simulink model "ES241A_MotAg2Meas"  (R2013b)
settings: Solver=FixedStepDiscrete  SolverMode=SingleTasking  StartTime=0.0  StopTime=1  FixedStep=0.002  RelTol=1e-3
undefined symbols (not defined in the file): ARCHGLBPRM_2PI_ULS_F32, FLTINJ_MOTAG2MEAS_MOTAG2MECL, MOTAG2ANSINCOSFLTFAILSTEP_CNT_U16, MOTAG2ANSINCOSFLTPASSSTEP_CNT_U16, MotAg2MeasOffs, MOTAG2MECLMAX_MOTREV_F32, MOTAG2MECLMIN_MOTREV_F32, NtcNr1, NtcSts1, sigbuilder_block, VALMAXERR_VOLTSQD_F32, VALMINERR_VOLTSQD_F32
libraries: simulink x12, NxtrLim x2, FloatToFixd x1, NxtrMath x1
(part 3 of 3)

== stateflow chart ES241A_MotAg2Meas/MotAg2Meas/MotAg2MeasPer1/MotPos_ArcTan/LimitMotAg2Meas/NormalizeMotAg2Mecl ==
  (default) -> (junction 3)
  (junction 3) -> (junction 5) : {MotAg2MeclVar=MotAg2MeclIn;}
  (junction 5) -> (junction 7) [order 2] : [MotAg2MeclVar<0]
  (junction 5) -> (junction 6) [order 1] : [MotAg2MeclVar>1]
  (junction 6) -> (junction 5) : {MotAg2MeclVar=MotAg2MeclVar-1;}
  (junction 7) -> (junction 5) : {MotAg2MeclVar=MotAg2MeclVar+1;}
  (junction 5) -> (junction 13) [order 3] : {MotAg2Mecl=MotAg2MeclVar;}
  data: MotAg2MeclIn input; MotAg2Mecl output single; MotAg2MeclVar local single

== stateflow chart ES241A_MotAg2Meas/MotAg2Meas/MotAg2MeasPer1/AnalogMsbDiagnostics/RollCnt_Qulfr_Calc/RollingCntr_Calc ==
  settings: stateMachineType=MEALY_MACHINE
  (default) -> (junction 4)
  (junction 4) -> (junction 6) [order 1] : [TestOk==1]
  (junction 6) -> (junction 36) [order 2] : {RollgCntr = PrevRollgCntr+1;}
  (junction 4) -> (junction 20) [order 2]
  (junction 6) -> (junction 36) [order 1] : [PrevRollgCntr == 255]
      | {
      | RollgCntr = 0;
      | }
  (junction 36) -> (junction 20)
  data: TestOk input; PrevRollgCntr input uint8 [0..255] =0; RollgCntr output uint8

== stateflow chart ES241A_MotAg2Meas/MotAg2Meas/MotAg2MeasPer1/AnalogMsbDiagnostics/RollCnt_Qulfr_Calc/SetNtcSts/ISO Fault Debounce Design ==
  note: NTCSTS_PASSD           (0)
      | NTCSTS_FAILD             (1)
      | NTCSTS_PREPASSD   (2)
      | NTCSTS_PREFAILD     (3)
      |
      | SIGQLFR_NORES        (0)
      | SIGQLFR_PASSD         (1)
      | SIGQLFR_FAILD           (2)
  note: Pass Loop
  note: Fail Loop
  note: 
  (default) -> (junction 89)
  (junction 89) -> (junction 95) [order 1] : [NtcSts ==3]
  (junction 89) -> (junction 93) [order 2] : [NtcSts ==2]
  (junction 89) -> (junction 141) [order 3] : [NtcSts ==1]
      | { ErrAcc = 32767;
      | Qualifier =2;
      |  }
  (junction 89) -> (junction 141) [order 4] : [NtcSts ==0]
      | { ErrAcc = -32768;
      | Qualifier=1;
      | }
  (junction 95) -> (junction 111) [order 1] : [ErrAcc <=0]
      | {ErrAcc = DebStep;}
  (junction 95) -> (junction 103) [order 2]
  (junction 93) -> (junction 123) [order 2] : {
      | ErrAcc = ErrAcc - DebStep;
      | }
  (junction 93) -> (junction 123) [order 1] : [(ErrAcc - DebStep) <= -32768]
      | {
      | ErrAcc = -32768;
      | Qualifier=1;
      | }
  (junction 103) -> (junction 111) [order 1] : [(ErrAcc + DebStep) <32767]
      | {ErrAcc = ErrAcc + DebStep;}
  (junction 103) -> (junction 111) [order 2] : {ErrAcc = 32767;
      | Qualifier =2;}
  (junction 123) -> (junction 141)
  (junction 111) -> (junction 141)
  (junction 141) -> (junction 159) [order 2] : {ErrAcc = 0;
      | Qualifier =0;
      | }
  (junction 141) -> (junction 159) [order 1] : [SvcClr ==0]
  data: NtcSts input uint8; Qualifier output uint8; DebStep input uint16; ErrAcc local int16; SvcClr input
